simulink model "singlephasefullwaveacvoltagecontroller"  (Simulink 7.3)
settings: Solver=ode23tb  StartTime=0.0  StopTime=0.1  MaxStep=1e-5  RelTol=1e-3
libraries: powerlib x9, powerlib_extras x2, simulink x1
settings Model: Creator=viswam  LastModifiedBy=viswam
settings SolverCC: InitialStep=1e-6
settings OptimizationCC: InitFltsAndDblsToZero=on
settings DebuggingCC: SaveWithParameterizedLinksMsg=none  SignalResolutionControl=TryResolveAllWithWarning  MultiTaskDSMMsg=warning  MultiTaskCondExecSysMsg=none
settings RTWCC: IncludeERTFirstTime=on
settings GRTTargetCC: TargetFcnLib=ansi_tfl_tmw.mat

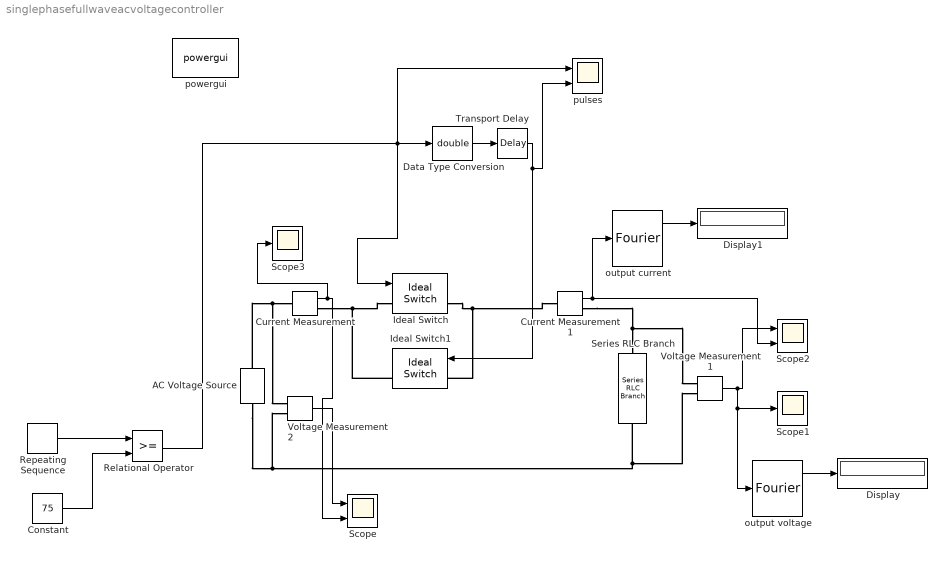
== system singlephasefullwaveacvoltagecontroller ==
  AC Voltage Source : powerlib/Electrical Sources/AC Voltage Source  DialogController=POWERSYS.PowerSysDialog  SystemSampleTime=-1  Amplitude=230*sqrt(2)  Phase=0  Frequency=50  SampleTime=0  Measurements=None
  Constant : Constant  Value=75  OutDataType=sfix(16)  OutScaling=2^0
  Current Measurement : powerlib/Measurements/Current Measurement  DialogController=POWERSYS.PowerSysDialog  SystemSampleTime=-1  PhasorSimulation=off  OutputType=Complex  PSBequivalent=0
  Current Measurement1 : powerlib/Measurements/Current Measurement  DialogController=POWERSYS.PowerSysDialog  SystemSampleTime=-1  PhasorSimulation=off  OutputType=Complex  PSBequivalent=0
  Data Type Conversion : DataTypeConversion  OutDataTypeMode=double  OutDataType=sfix(16)  OutScaling=2^0  OutDataTypeStr=double
  Display : Display
  Display1 : Display
  Ideal Switch : powerlib/Power Electronics/Ideal Switch  DialogController=POWERSYS.PowerSysDialog  SystemSampleTime=-1  Ron=0.001  Lon=0  IC=0  Rs=1e5  Cs=inf  Measurements=on
  Ideal Switch1 : powerlib/Power Electronics/Ideal Switch  DialogController=POWERSYS.PowerSysDialog  SystemSampleTime=-1  Ron=0.001  Lon=0  IC=0  Rs=1e5  Cs=inf  Measurements=on
  Relational Operator : RelationalOperator  LogicOutDataTypeMode=boolean  OutDataTypeStr=boolean
  Repeating Sequence : simulink/Sources/Repeating Sequence  SystemSampleTime=-1  rep_seq_t=[0 0.01 0.01 0.02]  rep_seq_y=[0 180 0 0]
  Scope : Scope  NumInputPorts=2
      settings: TimeRange=0.02  YMin=-400~-40  YMax=400~40
  Scope1 : Scope
      settings: TimeRange=0.02  YMin=-400  YMax=400  SaveName=outputvoltage  SampleInput=on  SampleTime=1e-6
  Scope2 : Scope  NumInputPorts=2
      settings: TimeRange=0.04  YMin=-400~-40  YMax=400~40  SaveName=ScopeData2
  Scope3 : Scope
      settings: TimeRange=0.02  YMin=-400  YMax=400  SaveName=inputcurrent  SampleInput=on  SampleTime=1e-6
  Series RLC Branch : powerlib/Elements/Series RLC Branch  DialogController=POWERSYS.PowerSysDialog  PhysicalDomain=powersysdomain  SubClassName=unknown  LeftPortType=p1  RightPortType=p1  LConnTagsString=__new0  RConnTagsString=__new0  BranchType=R  Resistance=10  Inductance=1e-3  SetiL0=off  InitialCurrent=0  Capacitance=1e-6  Setx0=off  InitialVoltage=0  Measurements=None
  Transport Delay : TransportDelay  DelayTime=0.01
  Voltage Measurement1 : powerlib/Measurements/Voltage Measurement  DialogController=POWERSYS.PowerSysDialog  SystemSampleTime=-1  PhasorSimulation=off  OutputType=Complex  PSBequivalent=0
  Voltage Measurement2 : powerlib/Measurements/Voltage Measurement  DialogController=POWERSYS.PowerSysDialog  SystemSampleTime=-1  PhasorSimulation=off  OutputType=Complex  PSBequivalent=0
  output current : powerlib_extras/Measurements/Fourier  DialogController=POWERSYS.PowerSysDialog  SystemSampleTime=-1  f1=50  n=1
  output voltage : powerlib_extras/Measurements/Fourier  DialogController=POWERSYS.PowerSysDialog  SystemSampleTime=-1  f1=50  n=1
  powergui : powerlib/powergui  Priority=1  SystemSampleTime=-1  SimulationMode=Continuous  SampleTime=50e-6  frequency=60  SPID=off  DisableSnubberDevices=off  DisableRonSwitches=off  DisableVfSwitches=off  SwTol=0  Interpol=off  frequencyindice=50  echomessages=off  HookPort=off  DisplayEquations=off  FunctionMessages=off  EnableUseOfTLC=off  x0status=blocks  RestoreLinks=warning  Frange=[0:2:500]  Ylog=off  Xlog=on  ShowGrid=off  save=off  variable=ZData  ZoomFFT=on  StartTime=0.0  cycles=1  DisplayStyle=1  fundamental=60  FreqAxis=off  MaxFrequency=1000  frequencyindicesteady=1  RmsSteady=1  display=off  Ts=0  methode=off
  pulses : Scope  NumInputPorts=2
      settings: TimeRange=0.02  YMin=-5~-5  YMax=5~5
  wires:
  Voltage Measurement2/1 -> Scope/1
  Current Measurement/1 -> Scope/2, Scope3/1
  Voltage Measurement1/1 -> Scope2/1, output voltage/1, Scope1/1
  Current Measurement1/1 -> Scope2/2, output current/1
  output voltage/1 -> Display/1
  output current/1 -> Display1/1
  Data Type Conversion/1 -> Transport Delay/1
  Transport Delay/1 -> pulses/2, Ideal Switch1/1
  Repeating Sequence/1 -> Relational Operator/1
  Constant/1 -> Relational Operator/2
  Relational Operator/1 -> Data Type Conversion/1, pulses/1, Ideal Switch/1
  connections:
  AC Voltage Source/RConn1 -- Current Measurement/LConn1 -- Voltage Measurement2/LConn1
  Ideal Switch1/RConn1 -- Current Measurement/RConn1 -- Ideal Switch/LConn1
  Ideal Switch1/LConn1 -- Current Measurement1/LConn1 -- Ideal Switch/RConn1
  Current Measurement1/RConn1 -- Series RLC Branch/LConn1 -- Voltage Measurement1/LConn1
  AC Voltage Source/LConn1 -- Series RLC Branch/RConn1 -- Voltage Measurement1/LConn2 -- Voltage Measurement2/LConn2
